simulink model "Tools"  (R2024b)
settings: Solver=ode45  StartTime=0.0  StopTime=10.0  RelTol=1e-3  EnableMultiTasking=on
values from neighbouring files (symbols this model uses):
  AAopti = [37.0 35.2 30.2 26.3 23.5 19.8 17.2 15.2 11.3 10.1  9.8  9.4  8.6  8.9  9.4 ... (first row only)    [InitISM_AII.m]
  Copti = [0.4 1.0 1.5 2.9 3.5 4.1 5.2 5.4 7.5  8.5  9.1  9.9 10.1 11.8 11.9 ... (first row only)    [InitISM_AII.m]
  gam = 1.4    [InitISM_AII.m]
  nv_remp = [0.090 0.110 0.120 0.110 0.130 0.150 0.135 0.155 0.140 0.145 0.140 0.135 0.120 0.120 ... (first row only)    [InitISM_AII.m]
  Pamb = 101300    [InitISM_AII.m]
  PRcrit = ((gam+1)/2)^(gam/(1-gam))    (= 0.528281787717)    [InitISM_AII.m]
  Rair = 287.0    (= 287)    [InitISM_AII.m]
  table_rdt_AA = [1.0000 0.9980 0.9955 0.9680 0.9500 0.9020 0.8195 0.6875 0.6080 0.5195 0.2000 0.0755]    [InitISM_AII.m]
  Tamb = 300    [InitISM_AII.m]
  vect_delta_AA = [0 2 3 8 10 14 19 25 28 31 40 43]    [InitISM_AII.m]
settings Model: Creator=Boanali  LastModifiedBy=ramse
settings DataIOCC: LimitDataPoints=on  SaveFormat=Array  SignalLoggingSaveFormat=ModelDataLogs  ReturnWorkspaceOutputs=off  SignalLoggingName=sigsOut
settings DebuggingCC: SaveWithParameterizedLinksMsg=none  UnderspecifiedInitializationDetection=Classic  MergeDetectMultiDrivingBlocksExec=none  SignalResolutionControl=TryResolveAllWithWarning  MultiTaskDSMMsg=warning  MultiTaskCondExecSysMsg=none  UnconnectedInputMsg=warning  UnconnectedOutputMsg=warning  UnconnectedLineMsg=warning
settings HardwareCC: ProdBitPerPointer=32  ProdBitPerSizeT=32  ProdBitPerPtrDiffT=32  ProdLargestAtomicFloat=None  ProdIntDivRoundTo=Undefined  ProdEndianess=Unspecified  ProdWordSize=32  ProdHWDeviceType=32-bit Generic  TargetUnknown=on
settings ModelReferenceCC: PropagateSignalLabelsOutOfModel=off
settings RTWCC: GPUComputeCapability=3.5
settings GRTTargetCC: CombineOutputUpdateFcns=off  GRTInterface=on
settings ConfigComp: CovMetricSettings=dw  CovSaveCumulativeToWorkspaceVar=on  CovSaveSingleToWorkspaceVar=on

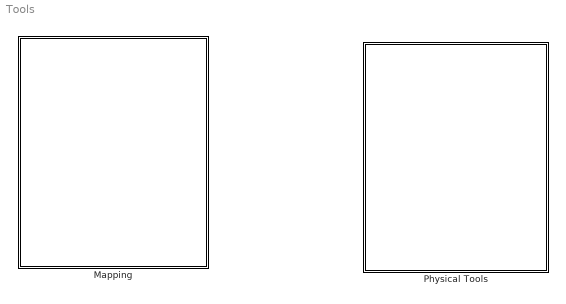
== system Tools ==
  Mapping : Subsystem
      mask Display: disp('CARTOGRAPHIES')
  Physical Tools : Subsystem
      mask Display: disp('PHYSICAL TOOLS')

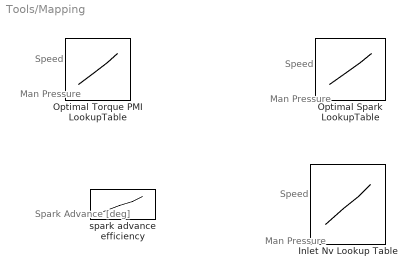
== system Tools/Mapping ==
  note: Speed
  note: Speed
  note: Spark Advance
      | [deg]
  note: Man Pressure
  note: Man Pressure
  note: Speed
  note: Man Pressure
  Inlet Nv Lookup Table : Lookup2D  RowIndex=Ne_remp  ColumnIndex=Pcol_remp  Table=nv_remp
  Optimal Spark LookupTable : Lookup2D  RowIndex=Ne_remp  ColumnIndex=Pcol_remp  Table=AAopti
  Optimal Torque PMI LookupTable : Lookup2D  RowIndex=Ne_remp  ColumnIndex=Pcol_remp  Table=Copti
  spark advance efficiency : Lookup  InputValues=vect_delta_AA  Table=table_rdt_AA

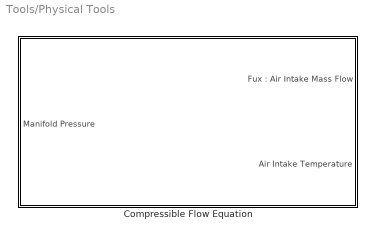
== system Tools/Physical Tools ==
  Compressible Flow Equation : Subsystem

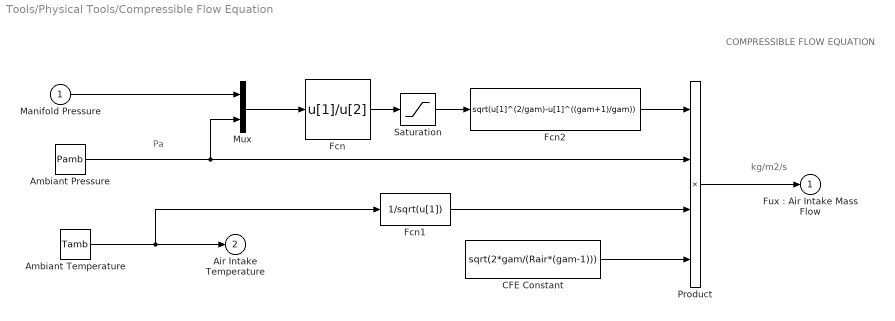
== system Tools/Physical Tools/Compressible Flow Equation ==
  note: COMPRESSIBLE FLOW EQUATION
  note: Pa
  note: kg/m2/s
  Manifold Pressure : Inport
  Ambiant Pressure : Constant  Value=Pamb
  Ambiant Temperature : Constant  Value=Tamb
  "CFE Constant " : Constant  Value=sqrt(2*gam/(Rair*(gam-1)))
  Fcn : Fcn  Expr=u[1]/u[2]
  Fcn1 : Fcn  Expr=1/sqrt(u[1])
  Fcn2 : Fcn  Expr=sqrt(u[1]^(2/gam)-u[1]^((gam+1)/gam))
  Mux : Mux  Inputs=2
  Product : Product  Inputs=4  InputSameDT=on  SaturateOnIntegerOverflow=on  OutDataTypeStr=Inherit: Same as first input
  Saturation : Saturate  UpperLimit=1  LowerLimit=PRcrit
  "Fux : Air Intake Mass Flow" : Outport
  Air Intake Temperature : Outport  Port=2
  wires:
  Ambiant Pressure/1 -> Product/2, Mux/2
  Product/1 -> "Fux : Air Intake Mass Flow"/1
  "CFE Constant "/1 -> Product/4
  Fcn2/1 -> Product/1
  Saturation/1 -> Fcn2/1
  Fcn1/1 -> Product/3
  Fcn/1 -> Saturation/1
  Mux/1 -> Fcn/1
  Manifold Pressure/1 -> Mux/1
  Ambiant Temperature/1 -> Fcn1/1, Air Intake Temperature/1
